simulink model "test_navigation3_0"  (R2017a)
settings: Solver=VariableStepAuto  StartTime=0.0  StopTime=inf  RelTol=1e-3
settings Model: Creator=xiaodong  LastModifiedBy=xiaodong

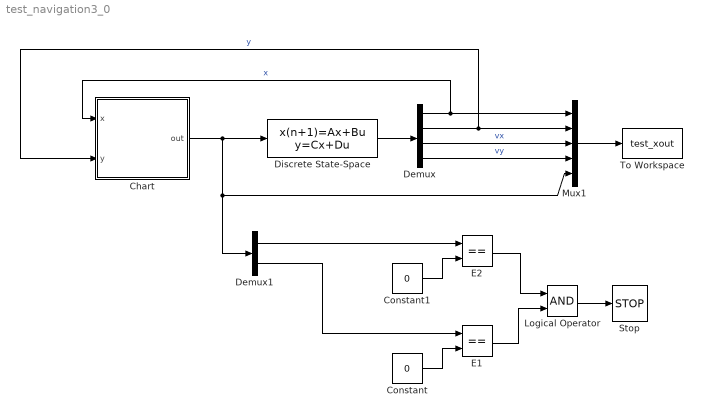
== system test_navigation3_0 ==
  Chart : Stateflow chart  TreatAsAtomicUnit=on
  Constant : Constant  Value=0
  Constant1 : Constant  Value=0
  Demux : Demux
  Demux1 : Demux  Outputs=2
  Discrete State-Space : DiscreteStateSpace  A=[1 0 0.01 0; 0 1 0 0.01; 0, 0, 0.9881, 0.0010; 0, 0, 0.0010, 0.9881]  B=[0 0; 0 0; 1 0; 0 1]  C=eye(4,4)  D=zeros(4,2)  X0="[1.60000000000000\t1.90000000000000\t-1.60000000000000\t0]"  SampleTime=-1
  E1 : RelationalOperator  Operator===  OutDataTypeStr=boolean  RndMeth=Simplest
  E2 : RelationalOperator  Operator===  OutDataTypeStr=boolean  RndMeth=Simplest
  Logical Operator : Logic  AllPortsSameDT=off  OutDataTypeStr=boolean
  Mux1 : Mux  Inputs=5
  Stop : Stop
  To Workspace : ToWorkspace  VariableName=test_xout  SampleTime=-1
  wires:
  Discrete State-Space/1 -> Demux/1
  Demux/4 -> Mux1/4  "vy"
  Demux/3 -> Mux1/3  "vx"
  Demux/1 -> Chart/1(x), Mux1/1  "x"
  Demux/2 -> Chart/2(y), Mux1/2  "y"
  Mux1/1 -> To Workspace/1
  Demux1/1 -> E2/1
  Constant1/1 -> E2/2
  Constant/1 -> E1/2
  E2/1 -> Logical Operator/1
  E1/1 -> Logical Operator/2
  Logical Operator/1 -> Stop/1
  Chart/1(out) -> Demux1/1, Mux1/5, Discrete State-Space/1
  Demux1/2 -> E1/1

== stateflow chart test_navigation3_0/Chart ==
  state s2
    entry:
    out = [0.0010;  -0.0119];
    during:
    out = [0.0010;  -0.0119];
  state s3
    entry:
    out = [0.0091;  -0.0091];
    during:
    out = [0.0091;  -0.0091];
  state s1
    entry:
    out = [0.0119;  -0.0010];
    during:
    out = [0.0119;  -0.0010];
  state s1_1
    entry:
    out = [0.0119;  -0.0010];
    during:
    out = [0.0119;  -0.0010];
  state s0
    entry:
    out = [0;  0];
    during:
    out = [0;  0];
  state s2_2
    entry:
    out = [0.0010;  -0.0119];
    during:
    out = [0.0010;  -0.0119];
  (default) -> s3
  s3 -> s2 [order 1] : [-0.9952*x-0.0072*y+1>0]
  s3 -> s1 [order 2] : [-0.0009*x-0.4984*y+1<0]
  s2 -> s1_1 : [-0.0036*x-1.0091*y+1>0]
  s3 -> s1_1 [order 4] : [-0.0073*x-1.0014*y+1>0]
  s3 -> s2_2 [order 3] : [-0.5003*x+0.0036*y+1<0]
  s1 -> s2_2 : [-0.4945*x-0.0021*y+1<0]
  s1_1 -> s0 : [-0.4990*x-0.0007*y+1<0]
  s2_2 -> s0 : [ 0.0026*x-1.0106*y+1>0]
  data: x input; y input; out output
